simulink model "Logging"  (R2018a)
settings: Solver=VariableStepAuto  StartTime=0.0  StopTime=10.0  RelTol=1e-3
PreLoadFcn:
  | modelDir = fileparts(get_param(bdroot, 'FileName'));
  | addpath(fullfile(modelDir,'../../Misc'));
undefined symbols (not defined in the file or in its folder): Ts
settings Model: Creator=Thomas  LastModifiedBy=Thomas
settings ModelReferenceCC: ModelReferenceNumInstancesAllowed=Single

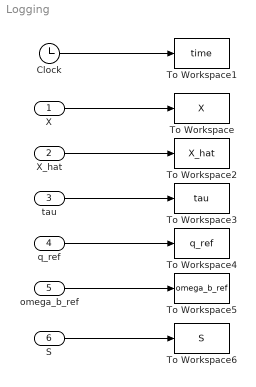
== system Logging ==
  X : Inport  PortDimensions=12
  X_hat : Inport  Port=2  PortDimensions=12
  tau : Inport  Port=3  PortDimensions=3
  q_ref : Inport  Port=4  PortDimensions=4
  omega_b_ref : Inport  Port=5  PortDimensions=3
  S : Inport  Port=6  PortDimensions=3
  Clock : Clock
  To Workspace : ToWorkspace  VariableName=X  SampleTime=Ts
  To Workspace1 : ToWorkspace  VariableName=time  SampleTime=Ts
  To Workspace2 : ToWorkspace  VariableName=X_hat  SampleTime=Ts
  To Workspace3 : ToWorkspace  VariableName=tau  SampleTime=Ts
  To Workspace4 : ToWorkspace  VariableName=q_ref  SampleTime=Ts
  To Workspace5 : ToWorkspace  VariableName=omega_b_ref  SampleTime=Ts
  To Workspace6 : ToWorkspace  VariableName=S  SampleTime=Ts
  wires:
  Clock/1 -> To Workspace1/1
  X/1 -> To Workspace/1
  X_hat/1 -> To Workspace2/1
  tau/1 -> To Workspace3/1
  q_ref/1 -> To Workspace4/1
  omega_b_ref/1 -> To Workspace5/1
  S/1 -> To Workspace6/1
